simulink model "Model"  (R2015b)
settings: Solver=ode45  StartTime=0.0  StopTime=1000  RelTol=1e-3
values from neighbouring files (symbols this model uses):
  center_xy = [6;0]    [script_backstepping.m]
  mu = 0.02    [script_backstepping.m]
  p0 = [7;0]    [script_backstepping.m]
  pd_0 = [2;0]    [script_backstepping.m]
  pd_1 = [10;4]    [script_backstepping.m]
  radii_xy = [5;3]    [script_backstepping.m]
  U_max = 0.1    [script_backstepping.m]
settings Model: Creator=shivjr  LastModifiedBy=Shiv Jeet rai
settings DataIOCC: SaveFormat=Array
settings HardwareCC: ProdBitPerPointer=32  ProdLargestAtomicFloat=None  ProdIntDivRoundTo=Undefined  ProdEndianess=Unspecified  ProdWordSize=32  ProdHWDeviceType=32-bit Generic
settings GRTTargetCC: GeneratePreprocessorConditionals=Disable all
settings ConfigComp: CovModelRefEnable=Off

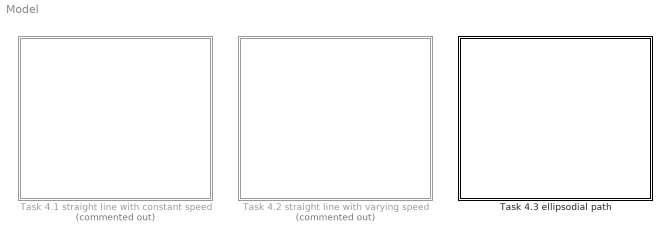
== system Model ==
  Task 4.1 straight line with constant speed : Subsystem  Commented=on
  Task 4.2 straight line with varying speed : Subsystem  Commented=on
  Task 4.3 ellipsodial path : Subsystem

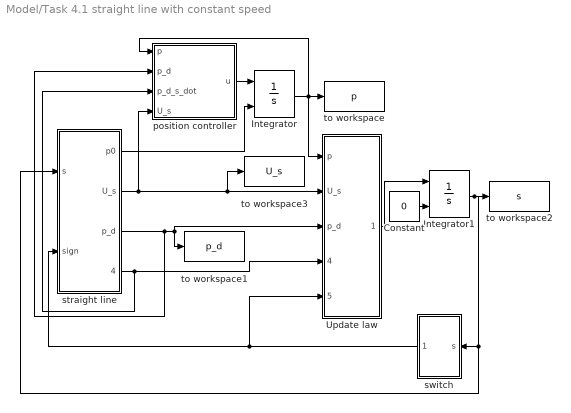
== system Model/Task 4.1 straight line with constant speed ==
  Constant : Constant  Value=0
  Integrator : Integrator  InitialConditionSource=external
  Integrator1 : Integrator  InitialConditionSource=external
  Update law : Subsystem
  position controller : Subsystem
  straight line : Subsystem
  switch : Subsystem
  to workspace : ToWorkspace  VariableName=p  SaveFormat=Timeseries  SampleTime=-1
  to workspace1 : ToWorkspace  VariableName=p_d  SaveFormat=Timeseries  SampleTime=-1
  to workspace2 : ToWorkspace  VariableName=s  SaveFormat=Timeseries  SampleTime=-1
  to workspace3 : ToWorkspace  VariableName=U_s  SaveFormat=Timeseries  SampleTime=-1
  wires:
  Integrator/1 -> Update law/1(p), to workspace/1, position controller/1(p)
  Update law/1(s_dot) -> Integrator1/1
  switch/1(sign) -> Update law/5(sigma), straight line/2(sign)
  straight line/4(p_d_s_dot) -> position controller/3(p_d_s_dot), Update law/4(p_d_s_dot)
  Constant/1 -> Integrator1/2
  position controller/1(u) -> Integrator/1
  straight line/3(p_d) -> position controller/2(p_d), to workspace1/1, Update law/3(p_d)
  straight line/1(p0) -> Integrator/2
  straight line/2(U_s) -> position controller/4(U_s), to workspace3/1, Update law/2(U_s)
  Integrator1/1 -> straight line/1(s), switch/1(s), to workspace2/1

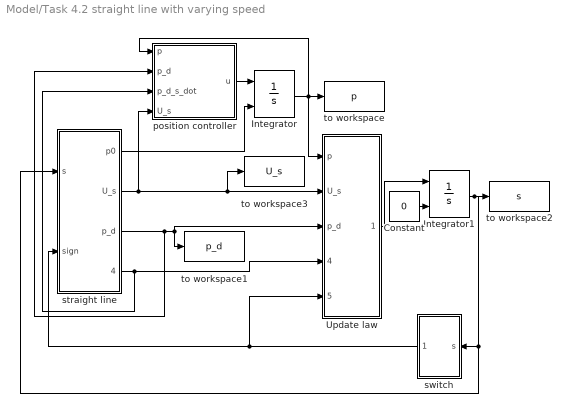
== system Model/Task 4.2 straight line with varying speed ==
  Constant : Constant  Value=0
  Integrator : Integrator  InitialConditionSource=external
  Integrator1 : Integrator  InitialConditionSource=external
  Update law : Subsystem
  position controller : Subsystem
  straight line : Subsystem
  switch : Subsystem
  to workspace : ToWorkspace  VariableName=p  SaveFormat=Timeseries  SampleTime=-1
  to workspace1 : ToWorkspace  VariableName=p_d  SaveFormat=Timeseries  SampleTime=-1
  to workspace2 : ToWorkspace  VariableName=s  SaveFormat=Timeseries  SampleTime=-1
  to workspace3 : ToWorkspace  VariableName=U_s  SaveFormat=Timeseries  SampleTime=-1
  wires:
  Integrator/1 -> Update law/1(p), to workspace/1, position controller/1(p)
  Update law/1(s_dot) -> Integrator1/1
  switch/1(sign) -> Update law/5(sigma), straight line/2(sign)
  straight line/4(p_d_s_dot) -> position controller/3(p_d_s_dot), Update law/4(p_d_s_dot)
  Constant/1 -> Integrator1/2
  position controller/1(u) -> Integrator/1
  straight line/3(p_d) -> position controller/2(p_d), to workspace1/1, Update law/3(p_d)
  straight line/1(p0) -> Integrator/2
  straight line/2(U_s) -> position controller/4(U_s), to workspace3/1, Update law/2(U_s)
  Integrator1/1 -> straight line/1(s), switch/1(s), to workspace2/1

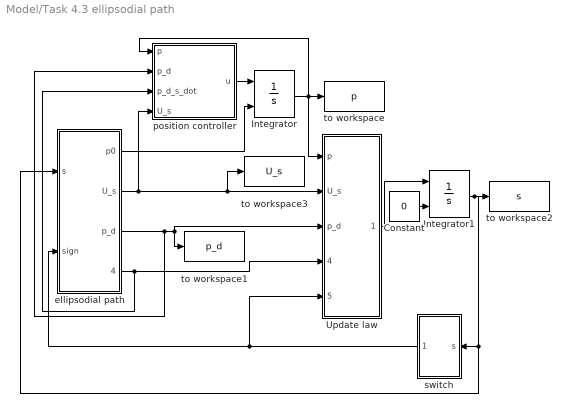
== system Model/Task 4.3 ellipsodial path ==
  Constant : Constant  Value=0
  Integrator : Integrator  InitialConditionSource=external
  Integrator1 : Integrator  InitialConditionSource=external
  Update law : Subsystem
  ellipsodial path : Subsystem
  position controller : Subsystem
  switch : Subsystem
  to workspace : ToWorkspace  VariableName=p  SaveFormat=Timeseries  SampleTime=-1
  to workspace1 : ToWorkspace  VariableName=p_d  SaveFormat=Timeseries  SampleTime=-1
  to workspace2 : ToWorkspace  VariableName=s  SaveFormat=Timeseries  SampleTime=-1
  to workspace3 : ToWorkspace  VariableName=U_s  SaveFormat=Timeseries  SampleTime=-1
  wires:
  Integrator/1 -> Update law/1(p), to workspace/1, position controller/1(p)
  Update law/1(s_dot) -> Integrator1/1
  switch/1(sign) -> Update law/5(sigma), ellipsodial path/2(sign)
  ellipsodial path/4(p_d_s_dot) -> position controller/3(p_d_s_dot), Update law/4(p_d_s_dot)
  Constant/1 -> Integrator1/2
  position controller/1(u) -> Integrator/1
  ellipsodial path/3(p_d) -> position controller/2(p_d), to workspace1/1, Update law/3(p_d)
  ellipsodial path/1(p0) -> Integrator/2
  ellipsodial path/2(U_s) -> position controller/4(U_s), to workspace3/1, Update law/2(U_s)
  Integrator1/1 -> ellipsodial path/1(s), switch/1(s), to workspace2/1

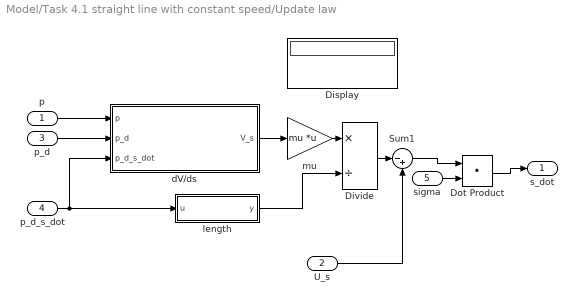
== system Model/Task 4.1 straight line with constant speed/Update law ==
  p : Inport
  U_s : Inport  Port=2
  p_d : Inport  Port=3
  p_d_s_dot : Inport  Port=4
  sigma : Inport  Port=5
  Display : Display
  Divide : Product  Inputs=*/
  Dot Product : DotProduct  InputSameDT=on  OutDataTypeStr=Inherit: Inherit via internal rule
  Sum1 : Sum  Inputs=|-+
  "dV/ds  " : MATLAB Function  TreatAsAtomicUnit=on
  length : MATLAB Function  TreatAsAtomicUnit=on
  mu : Gain  Gain=mu  Multiplication=Matrix(K*u)
  s_dot : Outport
  wires:
  p/1 -> "dV/ds  "/1(p)
  mu/1 -> Divide/1
  Divide/1 -> Sum1/1
  "dV/ds  "/1(V_s) -> mu/1
  p_d/1 -> "dV/ds  "/2(p_d)
  p_d_s_dot/1 -> "dV/ds  "/3(p_d_s_dot), length/1(u)
  length/1(y) -> Divide/2
  U_s/1 -> Sum1/2
  Sum1/1 -> Dot Product/1
  Dot Product/1 -> s_dot/1
  sigma/1 -> Dot Product/2

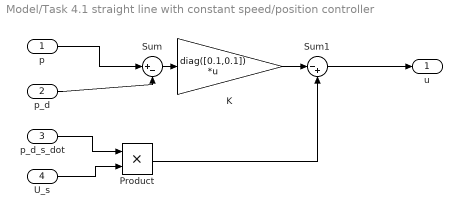
== system Model/Task 4.1 straight line with constant speed/position controller ==
  p : Inport
  p_d : Inport  Port=2
  p_d_s_dot : Inport  Port=3
  U_s : Inport  Port=4
  K : Gain  Gain=diag([0.1,0.1])  Multiplication=Matrix(K*u)
  Product : Product
  Sum : Sum  Inputs=|+-
  Sum1 : Sum  Inputs=|-+
  u : Outport
  wires:
  Sum/1 -> K/1
  p_d_s_dot/1 -> Product/1
  U_s/1 -> Product/2
  K/1 -> Sum1/1
  Product/1 -> Sum1/2
  Sum1/1 -> u/1
  p_d/1 -> Sum/2
  p/1 -> Sum/1

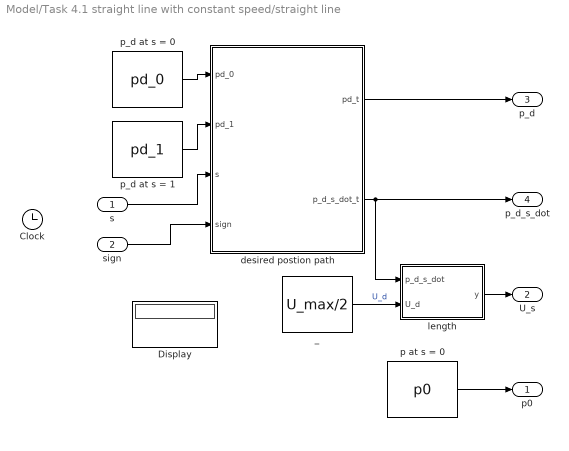
== system Model/Task 4.1 straight line with constant speed/straight line ==
  s : Inport
  sign : Inport  Port=2
  Clock : Clock
  Display : Display
  _ : Constant  Value=U_max/2
  desired postion path : MATLAB Function  TreatAsAtomicUnit=on
  length : MATLAB Function  TreatAsAtomicUnit=on
  p at s = 0 : Constant  Value=p0
  p_d at s = 0 : Constant  Value=pd_0
  p_d at s = 1 : Constant  Value=pd_1
  p0 : Outport
  U_s : Outport  Port=2
  p_d : Outport  Port=3
  p_d_s_dot : Outport  Port=4
  wires:
  p_d at s = 1/1 -> desired postion path/2(pd_1)
  p_d at s = 0/1 -> desired postion path/1(pd_0)
  desired postion path/1(pd_t) -> p_d/1
  p at s = 0/1 -> p0/1
  desired postion path/2(p_d_s_dot_t) -> length/1(p_d_s_dot), p_d_s_dot/1
  _/1 -> length/2(U_d)  "U_d"
  length/1(y) -> U_s/1
  s/1 -> desired postion path/3(s)
  sign/1 -> desired postion path/4(sign)

== system Model/Task 4.1 straight line with constant speed/switch ==
  s : Inport
  Memory : Memory  X0=1
  switch with respect to s : MATLAB Function  TreatAsAtomicUnit=on
  sign : Outport
  wires:
  switch with respect to s/1(sign_) -> sign/1, Memory/1
  Memory/1 -> switch with respect to s/2(prev_sign)
  s/1 -> switch with respect to s/1(s)

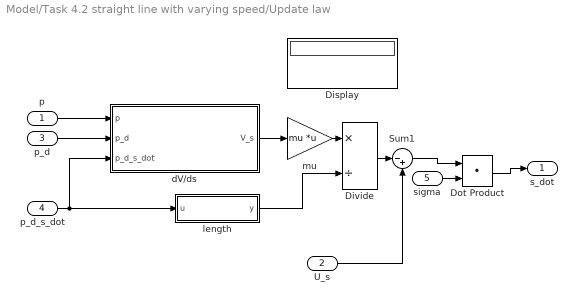
== system Model/Task 4.2 straight line with varying speed/Update law ==
  p : Inport
  U_s : Inport  Port=2
  p_d : Inport  Port=3
  p_d_s_dot : Inport  Port=4
  sigma : Inport  Port=5
  Display : Display
  Divide : Product  Inputs=*/
  Dot Product : DotProduct  InputSameDT=on  OutDataTypeStr=Inherit: Inherit via internal rule
  Sum1 : Sum  Inputs=|-+
  "dV/ds  " : MATLAB Function  TreatAsAtomicUnit=on
  length : MATLAB Function  TreatAsAtomicUnit=on
  mu : Gain  Gain=mu  Multiplication=Matrix(K*u)
  s_dot : Outport
  wires:
  p/1 -> "dV/ds  "/1(p)
  mu/1 -> Divide/1
  Divide/1 -> Sum1/1
  "dV/ds  "/1(V_s) -> mu/1
  p_d/1 -> "dV/ds  "/2(p_d)
  p_d_s_dot/1 -> "dV/ds  "/3(p_d_s_dot), length/1(u)
  length/1(y) -> Divide/2
  U_s/1 -> Sum1/2
  Sum1/1 -> Dot Product/1
  Dot Product/1 -> s_dot/1
  sigma/1 -> Dot Product/2

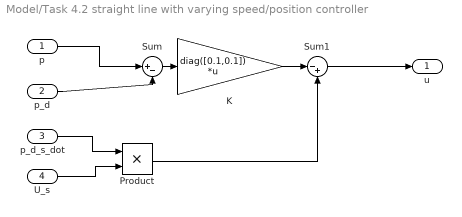
== system Model/Task 4.2 straight line with varying speed/position controller ==
  p : Inport
  p_d : Inport  Port=2
  p_d_s_dot : Inport  Port=3
  U_s : Inport  Port=4
  K : Gain  Gain=diag([0.1,0.1])  Multiplication=Matrix(K*u)
  Product : Product
  Sum : Sum  Inputs=|+-
  Sum1 : Sum  Inputs=|-+
  u : Outport
  wires:
  Sum/1 -> K/1
  p_d_s_dot/1 -> Product/1
  U_s/1 -> Product/2
  K/1 -> Sum1/1
  Product/1 -> Sum1/2
  Sum1/1 -> u/1
  p_d/1 -> Sum/2
  p/1 -> Sum/1

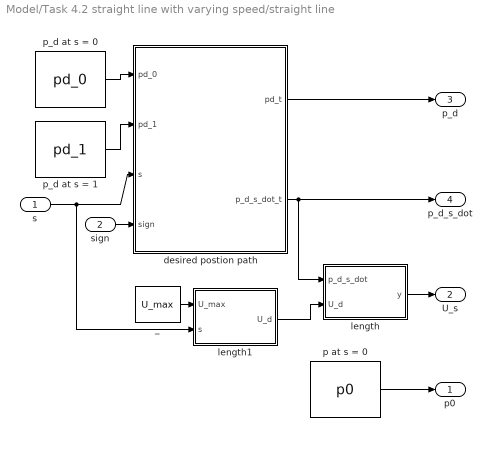
== system Model/Task 4.2 straight line with varying speed/straight line ==
  s : Inport
  sign : Inport  Port=2
  _ : Constant  Value=U_max
  desired postion path : MATLAB Function  TreatAsAtomicUnit=on
  length : MATLAB Function  TreatAsAtomicUnit=on
  length1 : MATLAB Function  TreatAsAtomicUnit=on
  p at s = 0 : Constant  Value=p0
  p_d at s = 0 : Constant  Value=pd_0
  p_d at s = 1 : Constant  Value=pd_1
  p0 : Outport
  U_s : Outport  Port=2
  p_d : Outport  Port=3
  p_d_s_dot : Outport  Port=4
  wires:
  p_d at s = 1/1 -> desired postion path/2(pd_1)
  p_d at s = 0/1 -> desired postion path/1(pd_0)
  desired postion path/1(pd_t) -> p_d/1
  p at s = 0/1 -> p0/1
  desired postion path/2(p_d_s_dot_t) -> length/1(p_d_s_dot), p_d_s_dot/1
  length/1(y) -> U_s/1
  s/1 -> length1/2(s), desired postion path/3(s)
  sign/1 -> desired postion path/4(sign)
  _/1 -> length1/1(U_max)
  length1/1(U_d) -> length/2(U_d)

== system Model/Task 4.2 straight line with varying speed/switch ==
  s : Inport
  Memory : Memory  X0=1
  switch with respect to s : MATLAB Function  TreatAsAtomicUnit=on
  sign : Outport
  wires:
  switch with respect to s/1(sign_) -> sign/1, Memory/1
  Memory/1 -> switch with respect to s/2(prev_sign)
  s/1 -> switch with respect to s/1(s)

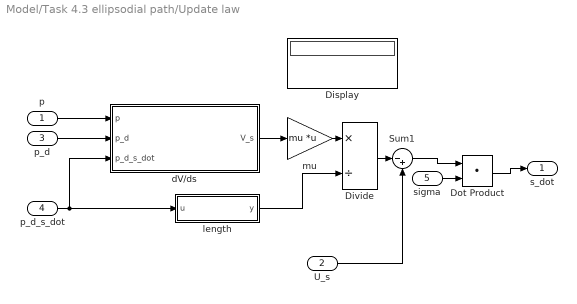
== system Model/Task 4.3 ellipsodial path/Update law ==
  p : Inport
  U_s : Inport  Port=2
  p_d : Inport  Port=3
  p_d_s_dot : Inport  Port=4
  sigma : Inport  Port=5
  Display : Display
  Divide : Product  Inputs=*/
  Dot Product : DotProduct  InputSameDT=on  OutDataTypeStr=Inherit: Inherit via internal rule
  Sum1 : Sum  Inputs=|-+
  "dV/ds  " : MATLAB Function  TreatAsAtomicUnit=on
  length : MATLAB Function  TreatAsAtomicUnit=on
  mu : Gain  Gain=mu  Multiplication=Matrix(K*u)
  s_dot : Outport
  wires:
  p/1 -> "dV/ds  "/1(p)
  mu/1 -> Divide/1
  Divide/1 -> Sum1/1
  "dV/ds  "/1(V_s) -> mu/1
  p_d/1 -> "dV/ds  "/2(p_d)
  p_d_s_dot/1 -> "dV/ds  "/3(p_d_s_dot), length/1(u)
  length/1(y) -> Divide/2
  U_s/1 -> Sum1/2
  Sum1/1 -> Dot Product/1
  Dot Product/1 -> s_dot/1
  sigma/1 -> Dot Product/2

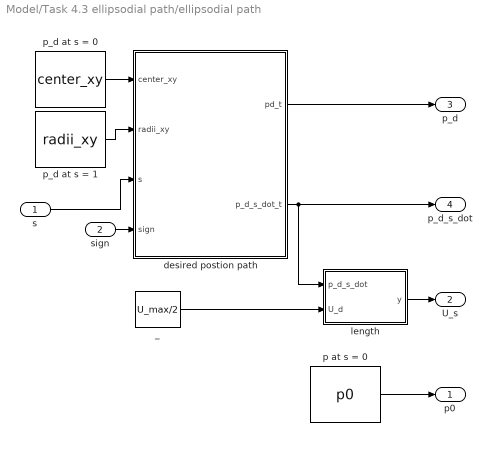
== system Model/Task 4.3 ellipsodial path/ellipsodial path ==
  s : Inport
  sign : Inport  Port=2
  _ : Constant  Value=U_max/2
  desired postion path : MATLAB Function  TreatAsAtomicUnit=on
  length : MATLAB Function  TreatAsAtomicUnit=on
  p at s = 0 : Constant  Value=p0
  p_d at s = 0 : Constant  Value=center_xy
  p_d at s = 1 : Constant  Value=radii_xy
  p0 : Outport
  U_s : Outport  Port=2
  p_d : Outport  Port=3
  p_d_s_dot : Outport  Port=4
  wires:
  p_d at s = 1/1 -> desired postion path/2(radii_xy)
  p_d at s = 0/1 -> desired postion path/1(center_xy)
  desired postion path/1(pd_t) -> p_d/1
  p at s = 0/1 -> p0/1
  desired postion path/2(p_d_s_dot_t) -> length/1(p_d_s_dot), p_d_s_dot/1
  length/1(y) -> U_s/1
  s/1 -> desired postion path/3(s)
  sign/1 -> desired postion path/4(sign)
  _/1 -> length/2(U_d)

== system Model/Task 4.3 ellipsodial path/position controller ==
  p : Inport
  p_d : Inport  Port=2
  p_d_s_dot : Inport  Port=3
  U_s : Inport  Port=4
  K : Gain  Gain=diag([0.1,0.1])  Multiplication=Matrix(K*u)
  Product : Product
  Sum : Sum  Inputs=|+-
  Sum1 : Sum  Inputs=|-+
  u : Outport
  wires:
  Sum/1 -> K/1
  p_d_s_dot/1 -> Product/1
  U_s/1 -> Product/2
  K/1 -> Sum1/1
  Product/1 -> Sum1/2
  Sum1/1 -> u/1
  p_d/1 -> Sum/2
  p/1 -> Sum/1

== system Model/Task 4.3 ellipsodial path/switch ==
  s : Inport
  Memory : Memory  X0=1
  switch with respect to s : MATLAB Function  TreatAsAtomicUnit=on
  sign : Outport
  wires:
  switch with respect to s/1(sign_) -> sign/1, Memory/1
  Memory/1 -> switch with respect to s/2(prev_sign)
  s/1 -> switch with respect to s/1(s)

== matlab function Model/Task 4.1 straight line with constant speed/Update law/length ==
  data: u input; y output
function y = fcn(u)

y = sqrt(u(1)^2 + u(2)^2);

== matlab function Model/Task 4.1 straight line with constant speed/Update law/dV//ds   ==
  data: p input; V_s output; p_d input; p_d_s_dot input
function V_s = fcn(p, p_d, p_d_s_dot)

temp = - transpose(p - p_d)*p_d_s_dot;
V_s = temp;

== matlab function Model/Task 4.1 straight line with constant speed/straight line/length ==
  data: p_d_s_dot input; y output; U_d input
function y = fcn(p_d_s_dot,U_d)

y = U_d/sqrt(p_d_s_dot(1)^2 + p_d_s_dot(2)^2);

== matlab function Model/Task 4.1 straight line with constant speed/straight line/desired postion path ==
  data: pd_0 input; pd_1 input; pd_t output; p_d_s_dot_t output; s input size=1; sign input size=1
function [pd_t,p_d_s_dot_t] = fcn(pd_0,pd_1,s, sign)

if s >= 1,
    s = 1;
end

p_d_s_dot_t = [ (pd_1(1)-pd_0(1))*sign; 
                (pd_1(2)-pd_0(2))*sign];

pd_t =  [(pd_1(1)-pd_0(1))*s + pd_0(1);
         (pd_1(2)-pd_0(2))*s + pd_0(2)];   
end

== matlab function Model/Task 4.2 straight line with varying speed/Update law/dV//ds   ==
  data: p input; V_s output; p_d input; p_d_s_dot input
function V_s = fcn(p, p_d, p_d_s_dot)

temp = - transpose(p - p_d)*p_d_s_dot;
V_s = temp;

== matlab function Model/Task 4.1 straight line with constant speed/switch/switch with respect to s ==
  data: s input; sign_ output; prev_sign input
function sign_ = fcn(s, prev_sign)

if s > 1 
    sign_ = -1;
elseif s <= 0
        sign_ = 1;
else
    sign_ = prev_sign;
end

== matlab function Model/Task 4.2 straight line with varying speed/Update law/length ==
  data: u input; y output
function y = fcn(u)

y = sqrt(u(1)^2 + u(2)^2);

== matlab function Model/Task 4.2 straight line with varying speed/straight line/desired postion path ==
  data: pd_0 input; pd_1 input; pd_t output; p_d_s_dot_t output; s input size=1; sign input size=1
function [pd_t,p_d_s_dot_t] = fcn(pd_0,pd_1,s, sign)

if s >= 1,
    s = 1;
end

p_d_s_dot_t = [ (pd_1(1)-pd_0(1))*sign; 
                (pd_1(2)-pd_0(2))*sign];

pd_t =  [(pd_1(1)-pd_0(1))*s + pd_0(1);
         (pd_1(2)-pd_0(2))*s + pd_0(2)];   
end

== matlab function Model/Task 4.2 straight line with varying speed/straight line/length ==
  data: p_d_s_dot input; y output; U_d input
function y = fcn(p_d_s_dot,U_d)

y = U_d/sqrt(p_d_s_dot(1)^2 + p_d_s_dot(2)^2);

== matlab function Model/Task 4.2 straight line with varying speed/switch/switch with respect to s ==
  data: s input; sign_ output; prev_sign input
function sign_ = fcn(s, prev_sign)

if s > 1 
    sign_ = -1;
elseif s <= 0
        sign_ = 1;
else
    sign_ = prev_sign;
end

== matlab function Model/Task 4.2 straight line with varying speed/straight line/length1 ==
  data: U_max input; U_d output; s input
function U_d = fcn(U_max,s)

if s > 1
    s = 1;
elseif s < 0
    s = 0;
end

U_d = U_max*(1.01 + sin(2*pi*s - pi/2))/2;

== matlab function Model/Task 4.3 ellipsodial path/Update law/dV//ds   ==
  data: p input; V_s output; p_d input; p_d_s_dot input
function V_s = fcn(p, p_d, p_d_s_dot)

temp = - transpose(p - p_d)*p_d_s_dot;
V_s = temp;

== matlab function Model/Task 4.3 ellipsodial path/Update law/length ==
  data: u input; y output
function y = fcn(u)

y = sqrt(u(1)^2 + u(2)^2);

== matlab function Model/Task 4.3 ellipsodial path/ellipsodial path/desired postion path ==
  data: center_xy input; radii_xy input; pd_t output; p_d_s_dot_t output; s input size=1; sign input size=1
function [pd_t,p_d_s_dot_t] = fcn(center_xy,radii_xy,s, sign)

% if s >= 1,
%     s = 1;
% end

p_d_s_dot_t = [ -2*pi*radii_xy(1)*sin(2*pi*s)*sign; 
                2*pi*radii_xy(2)*cos(2*pi*s)*sign];

pd_t =  [radii_xy(1)*cos(2*pi*s)+center_xy(1);
         radii_xy(2)*sin(2*pi*s)+center_xy(2)];   
end

== matlab function Model/Task 4.3 ellipsodial path/ellipsodial path/length ==
  data: p_d_s_dot input; y output; U_d input
function y = fcn(p_d_s_dot,U_d)

y = U_d/sqrt(p_d_s_dot(1)^2 + p_d_s_dot(2)^2);

== matlab function Model/Task 4.3 ellipsodial path/switch/switch with respect to s ==
  data: s input; sign_ output; prev_sign input
function sign_ = fcn(s, prev_sign)

if s > 1 
    sign_ = 1;%-1;
elseif s <= 0
        sign_ = 1;
else
    sign_ = prev_sign;
end
